simulink model "secOrdFilt_checkout"  (Simulink 9.2)
settings: Solver=FixedStepDiscrete  StartTime=0.0  StopTime=10  FixedStep=SIM_dt  RelTol=1e-3
undefined symbols (not defined in the file or in its folder): FILT
settings Model: Creator=coewal  LastModifiedBy=coewal
settings DataIOCC: LimitDataPoints=off  SaveFormat=Dataset  SignalLoggingSaveFormat=Dataset
settings OptimizationCC: LifeSpan=auto
settings DebuggingCC: UnderspecifiedInitializationDetection=Simplified  MergeDetectMultiDrivingBlocksExec=error  FcnCallInpInsideContextMsg=error  StateNameClashWarn=none  SFUnexpectedBacktrackingDiag=error  SFNoUnconditionalDefaultTransitionDiag=error  SFExecutionAtInitializationDiag=warning
settings HardwareCC: ProdBitPerPointer=64  ProdBitPerSizeT=64  ProdBitPerPtrDiffT=64  ProdLargestAtomicFloat=Float  ProdIntDivRoundTo=Zero  ProdEndianess=LittleEndian  ProdWordSize=64  ProdHWDeviceType=Intel->x86-64 (Windows64)
settings ModelReferenceCC: PropagateSignalLabelsOutOfModel=on
settings SFSimCC: SimUseLocalCustomCode=on
settings RTWCC: RTWUseLocalCustomCode=on
settings CodeAppCC: StateflowObjectComments=off
settings GRTTargetCC: TargetLangStandard=C99 (ISO)  GeneratePreprocessorConditionals=Use local settings  CombineOutputUpdateFcns=on  GRTInterface=off
settings ConfigComp: CovMetricSettings=dwe  CovHtmlReporting=off  CovSaveCumulativeToWorkspaceVar=off  CovSaveSingleToWorkspaceVar=off  CovExternalEMLEnable=on

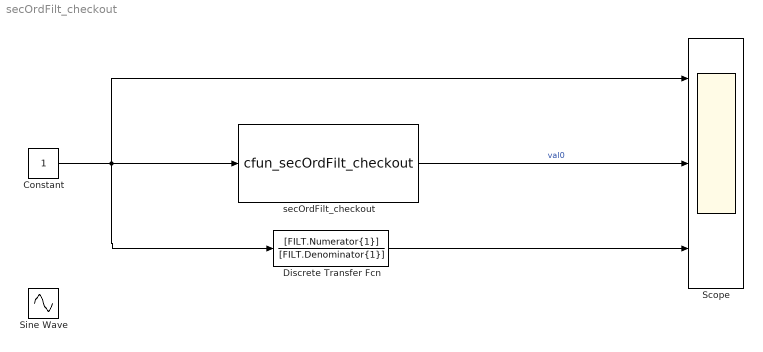
== system secOrdFilt_checkout ==
  Constant : Constant
  Discrete Transfer Fcn : DiscreteTransferFcn  Numerator=[FILT.Numerator{1}]  Denominator=[FILT.Denominator{1}]
  Scope : Scope  NumInputPorts=3
  Sine Wave : Sin  SampleTime=0
  secOrdFilt_checkout : S-Function  FunctionName=cfun_secOrdFilt_checkout  Parameters=SIM_dt, a0, a1, a2, b0, b1, b2  SFunctionDeploymentMode=off  EnableBusSupport=off
  wires:
  Constant/1 -> Scope/1, secOrdFilt_checkout/1, Discrete Transfer Fcn/1
  Discrete Transfer Fcn/1 -> Scope/3
  secOrdFilt_checkout/1 -> Scope/2  "val0"
